simulink model "Basic_cosimulation_circuit"  (R2021b)
settings: Solver=ode4  StartTime=0.0  StopTime=inf  FixedStep=Ts  RelTol=1e-3  EnableMultiTasking=on
PostLoadFcn:
  | %
  | % Script for validation of swtiching model design with it's respective
  | % average model.
  | %
  | % Here it is presented the design of the inverter to the 6 kW Fuel Cell
  | % model.
  | 
  | %%% Initialization %%%
  | 
  | 
  | % ------------------------------------- %
  | % ---------- Inverter Design ---------- %
  | % ------------------------------------- %
  | 
  | %%%% Nominal Parameters %%%%
  | 
  | Pnom = 50e3;                                        % Nominal Power
  | Vdc = 400;                                          % DC Voltage - Boost
  | m = 0.6;                                            % Modulation Index
  | Vnom_peak = m*Vdc/2;                                % Peak Voltage
  | Vnom_rms = Vnom_peak/sqrt(2);                       % Rms Voltage
  | FP_min = 0.9;                                       % For Reactive Power
  |                                                     % Compensation
  | Snom = Pnom/FP_min;                                 % Apparent Power
  | Irms = Pnom/(sqrt(3)*Vnom_rms);                     % Rms Curren
  | Inom_peak = Irms*sqrt(2);                           % Peak Current
  | Zbase = Vnom_peak/Inom_peak;                        % Base Impedance
  | f = 60;                                             % Nominal Frequency
  | wnom = 2*pi*60;                                     % Angular Frequency
  | 
  | % ------------------------- %
  | % Inverter LC Filter Design %
  | % ------------------------- %
  | 
  | fsw_inv = 96*60;                                    % Switching Frequency must be a multiple of the nominal frequency
  |                                                      % for proper operation of the Artemis Block
  | ripple_inv = 0.03;
  | L_inv = ((Vdc/2)-Vnom_peak)*(1/fsw_inv)/(ripple_inv*Inom_peak);
  | 
  | % - Capacitor
  | fres = 420;                                         % Filters Ressonant Frequency
  | 
  | Cf = 1/(4*L_inv*(pi^2)*(fres^2));                % Filter Capacitor
  | Rf = 1/(wnom*Cf*50);                                % Damping Resistor
  | 
  | % --- Sample Time --- %
  | 
  | Tsw = 0.00050;
  | Ts = Tsw/10;
  | 
  | % ---------------------- %
  | % Current Control Design %
  | % ---------------------- %
  | 
  | Ron = 0.001;                                        % IGBT Resistance
  | tau_i = 1e-3;                                       % Responde Time
  | kp_current = L_inv/tau_i;                           % PI Proportional Gain
  | ki_current = (Ron)/tau_i;                           % PI Integral Gain
  | 
  | decouple = (wnom*L_inv);                            % Decoupling Gain
InitFcn:
  | %
  | % Script for validation of swtiching model design with it's respective
  | % average model.
  | %
  | % Here it is presented the design of the inverter to the 6 kW Fuel Cell
  | % model.
  | 
  | %%% Initialization %%%
  | 
  | 
  | % ------------------------------------- %
  | % ---------- Inverter Design ---------- %
  | % ------------------------------------- %
  | 
  | %%%% Nominal Parameters %%%%
  | 
  | Pnom = 50e3;                                        % Nominal Power
  | Vdc = 400;                                          % DC Voltage - Boost
  | m = 0.6;                                            % Modulation Index
  | Vnom_peak = m*Vdc/2;                                % Peak Voltage
  | Vnom_rms = Vnom_peak/sqrt(2);                       % Rms Voltage
  | FP_min = 0.9;                                       % For Reactive Power
  |                                                     % Compensation
  | Snom = Pnom/FP_min;                                 % Apparent Power
  | Irms = Pnom/(sqrt(3)*Vnom_rms);                     % Rms Curren
  | Inom_peak = Irms*sqrt(2);                           % Peak Current
  | Zbase = Vnom_peak/Inom_peak;                        % Base Impedance
  | f = 60;                                             % Nominal Frequency
  | wnom = 2*pi*60;                                     % Angular Frequency
  | 
  | % ------------------------- %
  | % Inverter LC Filter Design %
  | % ------------------------- %
  | 
  | fsw_inv = 96*60;                                    % Switching Frequency must be a multiple of the nominal frequency
  |                                                      % for proper operation of the Artemis Block
  | ripple_inv = 0.03;
  | L_inv = ((Vdc/2)-Vnom_peak)*(1/fsw_inv)/(ripple_inv*Inom_peak);
  | 
  | % - Capacitor
  | fres = 420;                                         % Filters Ressonant Frequency
  | 
  | Cf = 1/(4*L_inv*(pi^2)*(fres^2));                % Filter Capacitor
  | Rf = 1/(wnom*Cf*50);                                % Damping Resistor
  | 
  | % --- Sample Time --- %
  | 
  | Tsw = 0.00050;
  | Ts = Tsw/10;
  | 
  | % ---------------------- %
  | % Current Control Design %
  | % ---------------------- %
  | 
  | Ron = 0.001;                                        % IGBT Resistance
  | tau_i = 1e-3;                                       % Responde Time
  | kp_current = L_inv/tau_i;                           % PI Proportional Gain
  | ki_current = (Ron)/tau_i;                           % PI Integral Gain
  | 
  | decouple = (wnom*L_inv);                            % Decoupling Gain
undefined symbols (not defined in the file or in its folder): D1, Delta, DiscIntNeverNeededParam, IP, j, ph, sps, UDP
libraries: spsCurrentMeasurementLib x25, spsControlledVoltageSourceLib x21, rtlab x18, spsGroundLib x13, spsThreePhaseSeriesRLCBranchLib x13, spsControlledCurrentSourceLib x11, spsVoltageMeasurementLib x10, simulink x8, rteventslib x8, powerlib_meascontrol x7, spsThreePhaseVIMeasurementLib x4, ssn_inverter_model x4
(part 5 of 5)

== system Basic_cosimulation_circuit/SM_Master/VSC_ITM_Average_Moving_Window/Control/Current Control/Inverse_Park_Transformation ==
  note: Park Transformation
  DQ : Inport
  Phase : Inport  Port=2
  Constant{1..4} (4 alike) : Constant  Value=2*pi/3
  Cos : Trigonometry  Operator=cos
  Cos1 : Trigonometry
  Cos2 : Trigonometry  Operator=cos
  Cos3 : Trigonometry
  Cos4 : Trigonometry  Operator=cos
  Cos5 : Trigonometry
  Demux : Demux  Outputs=2
  Gain : Gain  Gain=-1
  Gain1 : Gain  Gain=-1
  Gain2 : Gain  Gain=-1
  Mux : Mux  Inputs=3
  Product{,1..5} (6 alike) : Product
  Scope : Scope  NumInputPorts=2
  Sum1 : Sum
  Sum2 : Sum  Inputs=|+-
  Sum3 : Sum
  Sum4 : Sum  Inputs=|++
  Sum5 : Sum
  Sum6 : Sum  Inputs=|+-
  Sum7 : Sum  Inputs=|++
  ABC : Outport
  wires:
  Mux/1 -> Scope/2, ABC/1
  Sum1/1 -> [A]
  [phase] -> Cos1/1
  Product1/1 -> Sum1/2
  [Q] -> Product1/1
  Product/1 -> Sum1/1
  Cos/1 -> Product/2
  [phase] -> Cos/1
  [D] -> Product/1
  Phase/1 -> [phase]
  DQ/1 -> Scope/1, Demux/1
  Demux/1 -> [D]
  Demux/2 -> [Q]
  [D] -> Product2/1
  Cos2/1 -> Product2/2
  Product2/1 -> Sum3/1
  [Q] -> Product3/1
  Product3/1 -> Sum3/2
  [phase] -> Sum2/1
  Constant1/1 -> Sum2/2
  Sum2/1 -> Cos3/1
  Sum3/1 -> [B]
  Sum5/1 -> [C]
  [B] -> Mux/2
  [A] -> Mux/1
  [C] -> Mux/3
  Constant3/1 -> Sum6/2
  Sum6/1 -> Cos2/1
  [phase] -> Sum6/1
  [phase] -> Sum7/1
  Sum7/1 -> Cos4/1
  Constant4/1 -> Sum7/2
  Sum4/1 -> Cos5/1
  Constant2/1 -> Sum4/2
  [phase] -> Sum4/1
  Product5/1 -> Sum5/2
  [Q] -> Product5/1
  Product4/1 -> Sum5/1
  Cos4/1 -> Product4/2
  [D] -> Product4/1
  Cos1/1 -> Gain/1
  Cos3/1 -> Gain1/1
  Cos5/1 -> Gain2/1
  Gain/1 -> Product1/2
  Gain1/1 -> Product3/2
  Gain2/1 -> Product5/2

== system Basic_cosimulation_circuit/SM_Master/VSC_ITM_Instantaneous_values/Control/Current Control/Inverse_Park_Transformation ==
  note: Park Transformation
  DQ : Inport
  Phase : Inport  Port=2
  Constant{1..4} (4 alike) : Constant  Value=2*pi/3
  Cos : Trigonometry  Operator=cos
  Cos1 : Trigonometry
  Cos2 : Trigonometry  Operator=cos
  Cos3 : Trigonometry
  Cos4 : Trigonometry  Operator=cos
  Cos5 : Trigonometry
  Demux : Demux  Outputs=2
  Gain : Gain  Gain=-1
  Gain1 : Gain  Gain=-1
  Gain2 : Gain  Gain=-1
  Mux : Mux  Inputs=3
  Product{,1..5} (6 alike) : Product
  Scope : Scope  NumInputPorts=2
  Sum1 : Sum
  Sum2 : Sum  Inputs=|+-
  Sum3 : Sum
  Sum4 : Sum  Inputs=|++
  Sum5 : Sum
  Sum6 : Sum  Inputs=|+-
  Sum7 : Sum  Inputs=|++
  ABC : Outport
  wires:
  Mux/1 -> Scope/2, ABC/1
  Sum1/1 -> [A]
  [phase] -> Cos1/1
  Product1/1 -> Sum1/2
  [Q] -> Product1/1
  Product/1 -> Sum1/1
  Cos/1 -> Product/2
  [phase] -> Cos/1
  [D] -> Product/1
  Phase/1 -> [phase]
  DQ/1 -> Scope/1, Demux/1
  Demux/1 -> [D]
  Demux/2 -> [Q]
  [D] -> Product2/1
  Cos2/1 -> Product2/2
  Product2/1 -> Sum3/1
  [Q] -> Product3/1
  Product3/1 -> Sum3/2
  [phase] -> Sum2/1
  Constant1/1 -> Sum2/2
  Sum2/1 -> Cos3/1
  Sum3/1 -> [B]
  Sum5/1 -> [C]
  [B] -> Mux/2
  [A] -> Mux/1
  [C] -> Mux/3
  Constant3/1 -> Sum6/2
  Sum6/1 -> Cos2/1
  [phase] -> Sum6/1
  [phase] -> Sum7/1
  Sum7/1 -> Cos4/1
  Constant4/1 -> Sum7/2
  Sum4/1 -> Cos5/1
  Constant2/1 -> Sum4/2
  [phase] -> Sum4/1
  Product5/1 -> Sum5/2
  [Q] -> Product5/1
  Product4/1 -> Sum5/1
  Cos4/1 -> Product4/2
  [D] -> Product4/1
  Cos1/1 -> Gain/1
  Cos3/1 -> Gain1/1
  Cos5/1 -> Gain2/1
  Gain/1 -> Product1/2
  Gain1/1 -> Product3/2
  Gain2/1 -> Product5/2

== system Basic_cosimulation_circuit/SM_Master/VSC_ITM_SFA/Control/Current Control/Inverse_Park_Transformation ==
  note: Park Transformation
  DQ : Inport
  Phase : Inport  Port=2
  Constant{1..4} (4 alike) : Constant  Value=2*pi/3
  Cos : Trigonometry  Operator=cos
  Cos1 : Trigonometry
  Cos2 : Trigonometry  Operator=cos
  Cos3 : Trigonometry
  Cos4 : Trigonometry  Operator=cos
  Cos5 : Trigonometry
  Demux : Demux  Outputs=2
  Gain : Gain  Gain=-1
  Gain1 : Gain  Gain=-1
  Gain2 : Gain  Gain=-1
  Mux : Mux  Inputs=3
  Product{,1..5} (6 alike) : Product
  Scope : Scope  NumInputPorts=2
  Sum1 : Sum
  Sum2 : Sum  Inputs=|+-
  Sum3 : Sum
  Sum4 : Sum  Inputs=|++
  Sum5 : Sum
  Sum6 : Sum  Inputs=|+-
  Sum7 : Sum  Inputs=|++
  ABC : Outport
  wires:
  Mux/1 -> Scope/2, ABC/1
  Sum1/1 -> [A]
  [phase] -> Cos1/1
  Product1/1 -> Sum1/2
  [Q] -> Product1/1
  Product/1 -> Sum1/1
  Cos/1 -> Product/2
  [phase] -> Cos/1
  [D] -> Product/1
  Phase/1 -> [phase]
  DQ/1 -> Scope/1, Demux/1
  Demux/1 -> [D]
  Demux/2 -> [Q]
  [D] -> Product2/1
  Cos2/1 -> Product2/2
  Product2/1 -> Sum3/1
  [Q] -> Product3/1
  Product3/1 -> Sum3/2
  [phase] -> Sum2/1
  Constant1/1 -> Sum2/2
  Sum2/1 -> Cos3/1
  Sum3/1 -> [B]
  Sum5/1 -> [C]
  [B] -> Mux/2
  [A] -> Mux/1
  [C] -> Mux/3
  Constant3/1 -> Sum6/2
  Sum6/1 -> Cos2/1
  [phase] -> Sum6/1
  [phase] -> Sum7/1
  Sum7/1 -> Cos4/1
  Constant4/1 -> Sum7/2
  Sum4/1 -> Cos5/1
  Constant2/1 -> Sum4/2
  [phase] -> Sum4/1
  Product5/1 -> Sum5/2
  [Q] -> Product5/1
  Product4/1 -> Sum5/1
  Cos4/1 -> Product4/2
  [D] -> Product4/1
  Cos1/1 -> Gain/1
  Cos3/1 -> Gain1/1
  Cos5/1 -> Gain2/1
  Gain/1 -> Product1/2
  Gain1/1 -> Product3/2
  Gain2/1 -> Product5/2
